simulink model "DeratingControl"  (R2021b)
settings: Solver=VariableStepAuto  StartTime=0.0  StopTime=1  FixedStep=Ts  RelTol=1e-3
model workspace (MAT data in the model file):
  df = Simulink.Parameter
  df.Value = 0.9
  df.DataType = 'auto'
  df.Complexity = 'real'
  df.Dimensions = [1 1]
undefined symbols (not defined in the file): const_facInvTempDera, const_facMotTempDera, const_facPwrDera, const_SCD_tqDeraGenOvrd_C, const_stDera, const_tqBattDeraGenLim, const_tqBattDeraMotLim, const_tqDeraGen, const_tqDeraMot, const_tqDeraMotOvrd_C, const_tqEmMaxNp1, const_tqInvTempDeraMax, const_tqInvTempDeraMin, const_tqMotTempDeraMax, const_tqMotTempDeraMin, const_tqSpLim, const_tqSpLimMax, const_tqSpLimMin, const_tqTqReq
libraries: hdlsllib x10
settings Model: PacingRate=0.350000  Creator=win  LastModifiedBy=win

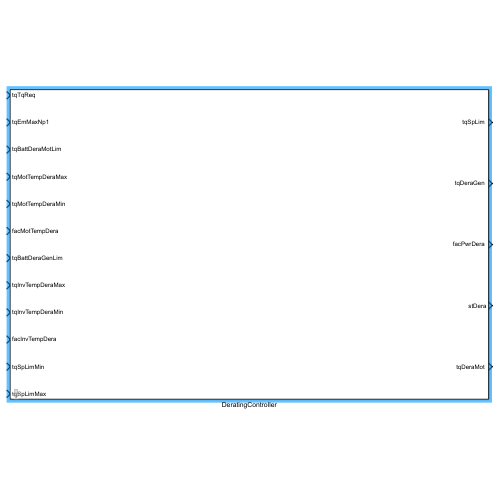
[thumbnail: Simulink's stored preview of the top-level diagram]
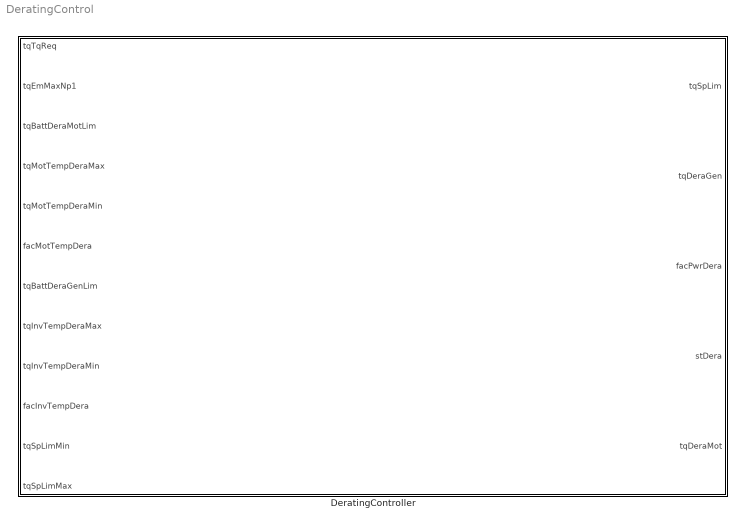
== system DeratingControl ==
  DeratingController : Subsystem  Description=Torque setpoint limit maximum value  mask{facGrdLimrUlim_C=5000, facGrdLimrLlim_C=-5000, bDeraMotOvrdActv_C=off, tqDeraMotOvrd_C=0, bDeraGenOvrdActv_C=off, SCD_tqDeraGenOvrd_C=0}
      mask prompts: facGrdLimrUlim_C "Gradient limiter upper factor"; facGrdLimrLlim_C "Gradient limiter lower factor"; bDeraMotOvrdActv_C "Motor mode derating override active"; tqDeraMotOvrd_C "Motor mode derating override torque"; bDeraGenOvrdActv_C "Generator mode derating override active"; SCD_tqDeraGenOvrd_C "Generator mode derating override torque"

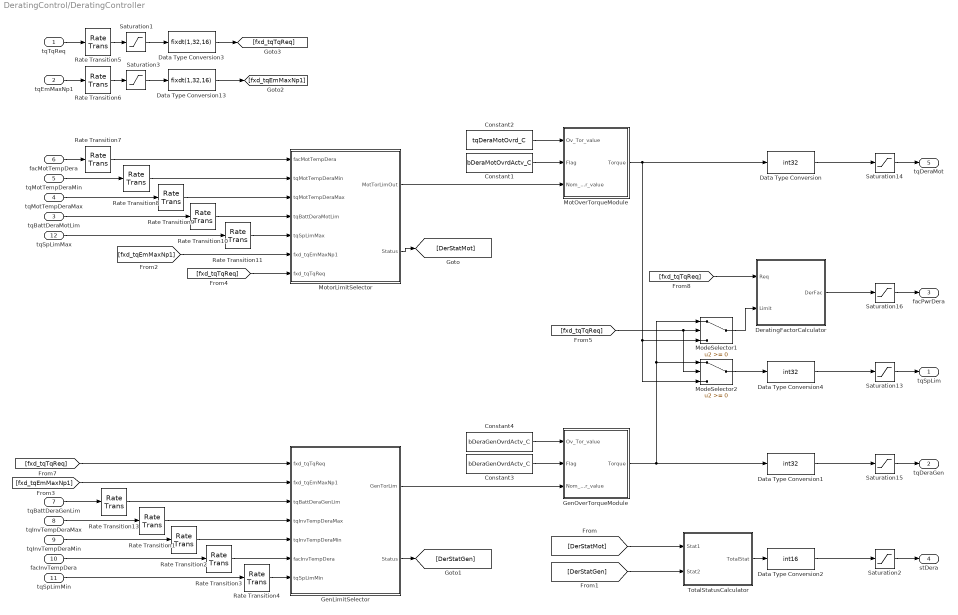
== system DeratingControl/DeratingController ==
  tqTqReq : Inport  Description=Torque request  OutMin=const_tqTqReq(1)  OutMax=const_tqTqReq(2)  OutDataTypeStr=int32
  tqEmMaxNp1 : Inport  Description=EM Maximum torque N+1 step  Port=2  OutMin=const_tqEmMaxNp1(1)  OutMax=const_tqEmMaxNp1(2)  OutDataTypeStr=int32
  tqBattDeraMotLim : Inport  Description=Derated motor mode torque output according to battery limits  Port=3  OutMin=const_tqBattDeraMotLim(1)  OutMax=const_tqBattDeraMotLim(2)  OutDataTypeStr=int32
  tqMotTempDeraMax : Inport  Description=Derated torque maximum value according to motor temperature  Port=4  OutMin=const_tqMotTempDeraMax(1)  OutMax=const_tqMotTempDeraMax(2)  OutDataTypeStr=int32
  tqMotTempDeraMin : Inport  Description=Derated torque minimum value according to motor temperature  Port=5  OutMin=const_tqMotTempDeraMin(1)  OutMax=const_tqMotTempDeraMin(2)  OutDataTypeStr=int32
  facMotTempDera : Inport  Description=Torque derating factor according to motor temperature  Port=6  OutMin=const_facMotTempDera(1)  OutMax=const_facMotTempDera(2)  OutDataTypeStr=int32
  tqBattDeraGenLim : Inport  Description=Derated generator mode torque output according to battery limits  Port=7  OutMin=const_tqBattDeraGenLim(1)  OutMax=const_tqBattDeraGenLim(2)  OutDataTypeStr=int32
  tqInvTempDeraMax : Inport  Description=Derated torque maximum value according to inverter temperature  Port=8  OutMin=const_tqInvTempDeraMax(1)  OutMax=const_tqInvTempDeraMax(2)  OutDataTypeStr=int32
  tqInvTempDeraMin : Inport  Description=Derated torque minimum value according to inverter temperature  Port=9  OutMin=const_tqInvTempDeraMin(1)  OutMax=const_tqInvTempDeraMin(2)  OutDataTypeStr=int32
  facInvTempDera : Inport  Description=Torque derating factor according to inverter temperature  Port=10  OutMin=const_facInvTempDera(1)  OutMax=const_facInvTempDera(2)  OutDataTypeStr=int32
  tqSpLimMin : Inport  Description=Torque setpoint limit minimum value  Port=11  OutMin=const_tqSpLimMin(1)  OutMax=const_tqSpLimMin(2)  OutDataTypeStr=int32
  tqSpLimMax : Inport  Description=Torque setpoint limit maximum value  Port=12  OutMin=const_tqSpLimMax(1)  OutMax=const_tqSpLimMax(2)  OutDataTypeStr=int32
  Constant1 : Constant  Value=bDeraMotOvrdActv_C
  Constant2 : Constant  Value=tqDeraMotOvrd_C
  Constant3 : Constant  Value=bDeraGenOvrdActv_C
  Constant4 : Constant  Value=bDeraGenOvrdActv_C
  Data Type Conversion : DataTypeConversion  OutDataTypeStr=int32
  Data Type Conversion1 : DataTypeConversion  OutDataTypeStr=int32
  Data Type Conversion13 : DataTypeConversion  OutDataTypeStr=fixdt(1,32,16)
  Data Type Conversion2 : DataTypeConversion  OutDataTypeStr=int16
  Data Type Conversion3 : DataTypeConversion  OutDataTypeStr=fixdt(1,32,16)
  Data Type Conversion4 : DataTypeConversion  OutDataTypeStr=int32
  DeratingFactorCalculator : Subsystem
  GenLimitSelector : Subsystem
  GenOverTorqueModule : Subsystem
  ModeSelector1 : Switch
  ModeSelector2 : Switch
  MotOverTorqueModule : Subsystem
  MotorLimitSelector : Subsystem
  Rate Transition{1..11,13} (12 alike) : RateTransition  OutPortSampleTime=Ts
  Saturation1 : Saturate  UpperLimit=const_tqTqReq(2)  LowerLimit=const_tqTqReq(1)
  Saturation13 : Saturate  UpperLimit=const_tqSpLim(2)  LowerLimit=const_tqSpLim(1)  OutDataTypeStr=int32
  Saturation14 : Saturate  UpperLimit=const_tqDeraMot(2)  LowerLimit=const_tqDeraMot(1)
  Saturation15 : Saturate  UpperLimit=const_tqDeraGen(2)  LowerLimit=const_tqDeraGen(1)
  Saturation16 : Saturate  UpperLimit=const_facPwrDera(2)  LowerLimit=const_facPwrDera(1)
  Saturation2 : Saturate  UpperLimit=const_stDera(2)  LowerLimit=const_stDera(1)  OutDataTypeStr=int32
  Saturation3 : Saturate  UpperLimit=const_tqEmMaxNp1(2)  LowerLimit=const_tqEmMaxNp1(1)
  TotalStatusCalculator : Subsystem
  "tqSpLim " : Outport  Description=Limited torque setpoint  OutMin=const_tqSpLim(1)  OutMax=const_tqSpLim(2)
  "tqDeraGen " : Outport  Description=Derated torque for generator mode  Port=2  OutMin=const_tqDeraGen(1)  OutMax=const_tqDeraGen(2)
  "facPwrDera " : Outport  Description=Power derating factor  Port=3  OutMin=const_facPwrDera(1)  OutMax=const_facPwrDera(2)
  stDera : Outport  Description=Derating status  Port=4
  "tqDeraMot " : Outport  Description=Derated torque for motor mode  Port=5
  wires:
  Saturation13/1 -> "tqSpLim "/1
  Saturation16/1 -> "facPwrDera "/1
  facMotTempDera/1 -> Rate Transition7/1
  tqMotTempDeraMin/1 -> Rate Transition8/1
  tqMotTempDeraMax/1 -> Rate Transition9/1
  tqBattDeraMotLim/1 -> Rate Transition10/1
  tqBattDeraGenLim/1 -> Rate Transition13/1
  tqInvTempDeraMax/1 -> Rate Transition1/1
  tqInvTempDeraMin/1 -> Rate Transition2/1
  facInvTempDera/1 -> Rate Transition3/1
  Constant4/1 -> GenOverTorqueModule/1(Ov_Tor_value)
  Constant3/1 -> GenOverTorqueModule/2(Flag)
  Constant2/1 -> MotOverTorqueModule/1(Ov_Tor_value)
  Constant1/1 -> MotOverTorqueModule/2(Flag)
  MotorLimitSelector/1(MotTorLimOut) -> MotOverTorqueModule/3(Nom_Tor_value)
  GenLimitSelector/1(GenTorLim) -> GenOverTorqueModule/3(Nom_Tor_value)
  Saturation15/1 -> "tqDeraGen "/1
  MotorLimitSelector/2(Status) -> [DerStatMot]
  GenOverTorqueModule/1(Torque) -> ModeSelector1/1, ModeSelector2/1, Data Type Conversion1/1
  GenLimitSelector/2(Status) -> [DerStatGen]
  [DerStatMot] -> TotalStatusCalculator/1(Stat1)
  [DerStatGen] -> TotalStatusCalculator/2(Stat2)
  Saturation2/1 -> stDera/1
  MotOverTorqueModule/1(Torque) -> ModeSelector2/3, ModeSelector1/3, Data Type Conversion/1
  tqSpLimMin/1 -> Rate Transition4/1
  tqSpLimMax/1 -> Rate Transition11/1
  ModeSelector2/1 -> Data Type Conversion4/1
  Saturation1/1 -> Data Type Conversion3/1
  Saturation3/1 -> Data Type Conversion13/1
  tqTqReq/1 -> Rate Transition5/1
  tqEmMaxNp1/1 -> Rate Transition6/1
  Rate Transition13/1 -> GenLimitSelector/3(tqBattDeraGenLim)
  Rate Transition1/1 -> GenLimitSelector/4(tqInvTempDeraMax)
  Rate Transition2/1 -> GenLimitSelector/5(tqInvTempDeraMin)
  Rate Transition3/1 -> GenLimitSelector/6("facInvTempDera ")
  Rate Transition4/1 -> GenLimitSelector/7("tqSpLimMin ")
  Rate Transition6/1 -> Saturation3/1
  Rate Transition5/1 -> Saturation1/1
  Rate Transition7/1 -> MotorLimitSelector/1("facMotTempDera ")
  Rate Transition8/1 -> MotorLimitSelector/2("tqMotTempDeraMin ")
  Rate Transition9/1 -> MotorLimitSelector/3("tqMotTempDeraMax ")
  Rate Transition10/1 -> MotorLimitSelector/4(tqBattDeraMotLim)
  Rate Transition11/1 -> MotorLimitSelector/5("tqSpLimMax ")
  Data Type Conversion13/1 -> [fxd_tqEmMaxNp1]
  [fxd_tqEmMaxNp1] -> MotorLimitSelector/6(fxd_tqEmMaxNp1)
  [fxd_tqEmMaxNp1] -> GenLimitSelector/2(fxd_tqEmMaxNp1)
  [fxd_tqTqReq] -> MotorLimitSelector/7(fxd_tqTqReq)
  Data Type Conversion3/1 -> [fxd_tqTqReq]
  [fxd_tqTqReq] -> ModeSelector2/2, ModeSelector1/2
  [fxd_tqTqReq] -> GenLimitSelector/1(fxd_tqTqReq)
  Data Type Conversion/1 -> Saturation14/1
  Saturation14/1 -> "tqDeraMot "/1
  Data Type Conversion1/1 -> Saturation15/1
  [fxd_tqTqReq] -> DeratingFactorCalculator/1(Req)
  ModeSelector1/1 -> DeratingFactorCalculator/2(Limit)
  DeratingFactorCalculator/1(DerFac) -> Saturation16/1
  Data Type Conversion4/1 -> Saturation13/1
  TotalStatusCalculator/1(TotalStat) -> Data Type Conversion2/1
  Data Type Conversion2/1 -> Saturation2/1

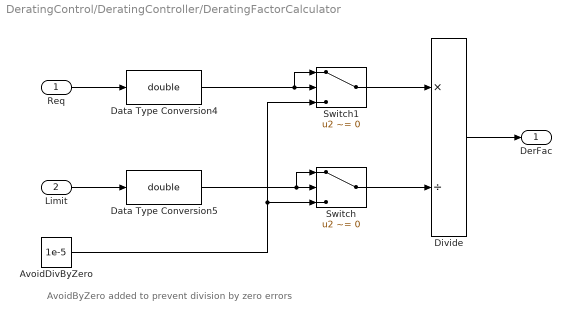
== system DeratingControl/DeratingController/DeratingFactorCalculator ==
  note: AvoidByZero added to prevent division by zero errors
  Req : Inport
  Limit : Inport  Port=2
  AvoidDivByZero : Constant  Value=1e-5  OutDataTypeStr=Inherit: Inherit via back propagation
  Data Type Conversion4 : DataTypeConversion  OutDataTypeStr=double
  Data Type Conversion5 : DataTypeConversion  OutDataTypeStr=double
  Divide : Product  Inputs=*/
  Switch : Switch  Criteria=u2 ~= 0  Threshold=1e-4
  Switch1 : Switch  Criteria=u2 ~= 0  Threshold=1e-4
  DerFac : Outport
  wires:
  Divide/1 -> DerFac/1
  Req/1 -> Data Type Conversion4/1
  Limit/1 -> Data Type Conversion5/1
  Data Type Conversion5/1 -> Switch/2, Switch/1
  Switch/1 -> Divide/2
  AvoidDivByZero/1 -> Switch/3, Switch1/3
  Switch1/1 -> Divide/1
  Data Type Conversion4/1 -> Switch1/2, Switch1/1

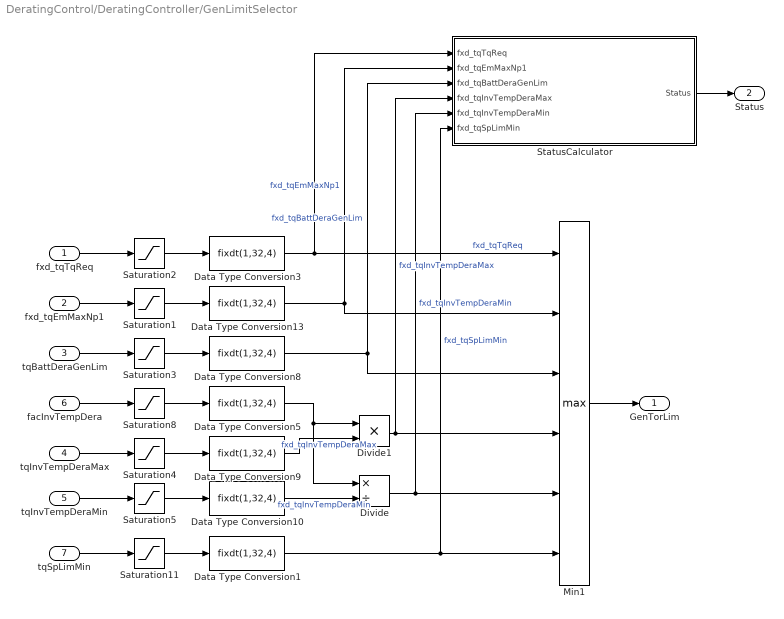
== system DeratingControl/DeratingController/GenLimitSelector ==
  fxd_tqTqReq : Inport
  fxd_tqEmMaxNp1 : Inport  Port=2
  tqBattDeraGenLim : Inport  Description=Derated generator mode torque output according to battery limits  Port=3  OutMin=const_tqBattDeraGenLim(1)  OutMax=const_tqBattDeraGenLim(2)  OutDataTypeStr=int32
  tqInvTempDeraMax : Inport  Description=Derated torque maximum value according to inverter temperature  Port=4  OutMin=const_tqInvTempDeraMax(1)  OutMax=const_tqInvTempDeraMax(2)  OutDataTypeStr=int32
  tqInvTempDeraMin : Inport  Description=Derated torque minimum value according to inverter temperature  Port=5  OutMin=const_tqInvTempDeraMin(1)  OutMax=const_tqInvTempDeraMin(2)  OutDataTypeStr=int32
  "facInvTempDera " : Inport  Description=Torque derating factor according to inverter temperature  Port=6  OutMin=const_facInvTempDera(1)  OutMax=const_facInvTempDera(2)  OutDataTypeStr=int32
  "tqSpLimMin " : Inport  Port=7
  Data Type Conversion{1,3,5,8..10,13} (7 alike) : DataTypeConversion  OutDataTypeStr=fixdt(1,32,4)
  Divide : Product  Inputs=*/
  Divide1 : Product  Inputs=**
  Min1 : MinMax  Function=max  Inputs=6
  Saturation1 : Saturate  UpperLimit=const_tqEmMaxNp1(2)  LowerLimit=const_tqEmMaxNp1(1)  OutDataTypeStr=double
  Saturation11 : Saturate  UpperLimit=const_tqSpLimMin(2)  LowerLimit=const_tqSpLimMin(1)  OutDataTypeStr=int32
  Saturation2 : Saturate  UpperLimit=const_tqTqReq(2)  LowerLimit=const_tqTqReq(1)  OutDataTypeStr=fixdt(1,32,12)
  Saturation3 : Saturate  UpperLimit=const_tqBattDeraGenLim(2)  LowerLimit=const_tqBattDeraGenLim(1)
  Saturation4 : Saturate  UpperLimit=const_tqInvTempDeraMax(2)  LowerLimit=const_tqInvTempDeraMax(1)  OutDataTypeStr=int32
  Saturation5 : Saturate  UpperLimit=const_tqInvTempDeraMin(2)  LowerLimit=const_tqInvTempDeraMin(1)  OutDataTypeStr=int32
  Saturation8 : Saturate  UpperLimit=1  LowerLimit=0  OutDataTypeStr=int32
  StatusCalculator : Subsystem
  GenTorLim : Outport
  Status : Outport  Port=2
  wires:
  Divide1/1 -> StatusCalculator/4(fxd_tqInvTempDeraMax), Min1/4  "fxd_tqInvTempDeraMax"
  Data Type Conversion8/1 -> Min1/3, StatusCalculator/3(fxd_tqBattDeraGenLim)  "fxd_tqBattDeraGenLim"
  Divide/1 -> StatusCalculator/5(fxd_tqInvTempDeraMin), Min1/5  "fxd_tqInvTempDeraMin"
  Saturation8/1 -> Data Type Conversion5/1
  Saturation4/1 -> Data Type Conversion9/1
  fxd_tqEmMaxNp1/1 -> Saturation1/1
  fxd_tqTqReq/1 -> Saturation2/1
  Saturation3/1 -> Data Type Conversion8/1
  Min1/1 -> GenTorLim/1
  "facInvTempDera "/1 -> Saturation8/1
  tqBattDeraGenLim/1 -> Saturation3/1
  tqInvTempDeraMax/1 -> Saturation4/1
  Saturation5/1 -> Data Type Conversion10/1
  tqInvTempDeraMin/1 -> Saturation5/1
  StatusCalculator/1(Status) -> Status/1
  Data Type Conversion13/1 -> Min1/2, StatusCalculator/2(fxd_tqEmMaxNp1)  "fxd_tqEmMaxNp1"
  Saturation1/1 -> Data Type Conversion13/1
  Data Type Conversion3/1 -> StatusCalculator/1(fxd_tqTqReq), Min1/1  "fxd_tqTqReq"
  Saturation2/1 -> Data Type Conversion3/1
  Saturation11/1 -> Data Type Conversion1/1
  Data Type Conversion1/1 -> Min1/6, StatusCalculator/6(fxd_tqSpLimMin)  "fxd_tqSpLimMin"
  "tqSpLimMin "/1 -> Saturation11/1
  Data Type Conversion10/1 -> Divide/2  "fxd_tqInvTempDeraMin"
  Data Type Conversion5/1 -> Divide/1, Divide1/1
  Data Type Conversion9/1 -> Divide1/2  "fxd_tqInvTempDeraMax"

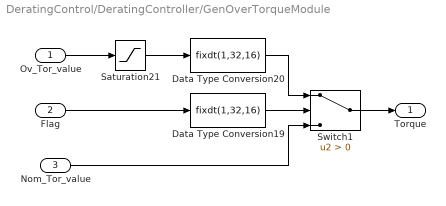
== system DeratingControl/DeratingController/GenOverTorqueModule ==
  Ov_Tor_value : Inport
  Flag : Inport  Port=2
  Nom_Tor_value : Inport  Port=3
  Data Type Conversion19 : DataTypeConversion  OutDataTypeStr=fixdt(1,32,16)
  Data Type Conversion20 : DataTypeConversion  OutDataTypeStr=fixdt(1,32,16)
  Saturation21 : Saturate  UpperLimit=const_SCD_tqDeraGenOvrd_C(2)  LowerLimit=const_SCD_tqDeraGenOvrd_C(1)  OutDataTypeStr=int32
  Switch1 : Switch  Criteria=u2 > Threshold  OutDataTypeStr=fixdt(1,32,16)
  Torque : Outport
  wires:
  Flag/1 -> Data Type Conversion19/1
  Saturation21/1 -> Data Type Conversion20/1
  Ov_Tor_value/1 -> Saturation21/1
  Data Type Conversion20/1 -> Switch1/1
  Data Type Conversion19/1 -> Switch1/2
  Switch1/1 -> Torque/1
  Nom_Tor_value/1 -> Switch1/3

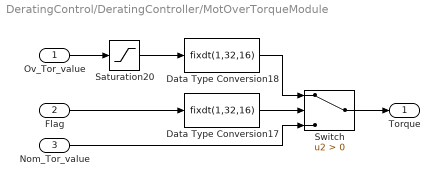
== system DeratingControl/DeratingController/MotOverTorqueModule ==
  Ov_Tor_value : Inport
  Flag : Inport  Port=2
  Nom_Tor_value : Inport  Port=3
  Data Type Conversion17 : DataTypeConversion  OutDataTypeStr=fixdt(1,32,16)
  Data Type Conversion18 : DataTypeConversion  OutDataTypeStr=fixdt(1,32,16)
  Saturation20 : Saturate  UpperLimit=const_tqDeraMotOvrd_C(2)  LowerLimit=const_tqDeraMotOvrd_C(1)  OutDataTypeStr=int32
  Switch : Switch  Criteria=u2 > Threshold  OutDataTypeStr=fixdt(1,32,16)
  Torque : Outport
  wires:
  Ov_Tor_value/1 -> Saturation20/1
  Saturation20/1 -> Data Type Conversion18/1
  Switch/1 -> Torque/1
  Data Type Conversion17/1 -> Switch/2
  Nom_Tor_value/1 -> Switch/3
  Data Type Conversion18/1 -> Switch/1
  Flag/1 -> Data Type Conversion17/1

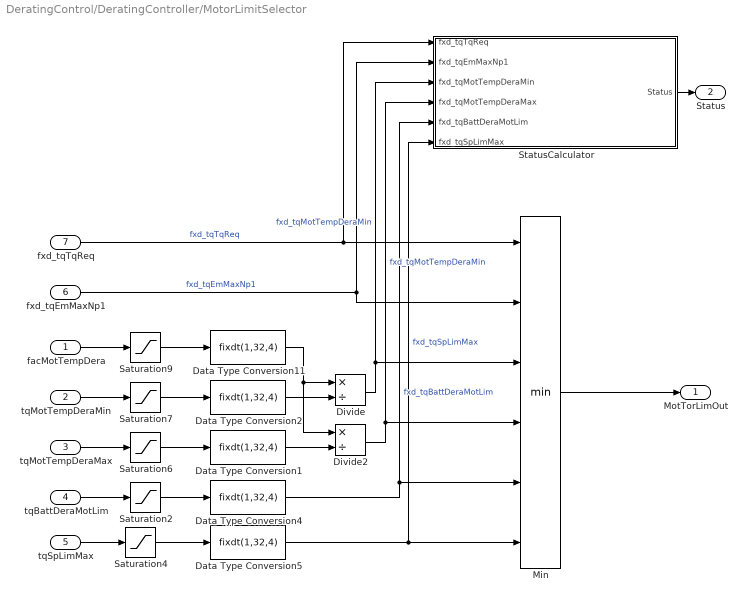
== system DeratingControl/DeratingController/MotorLimitSelector ==
  "facMotTempDera " : Inport  Description=Torque derating factor according to motor temperature  OutMin=const_facMotTempDera(1)  OutMax=const_facMotTempDera(2)  OutDataTypeStr=int32
  "tqMotTempDeraMin " : Inport  Description=Derated torque minimum value according to motor temperature  Port=2  OutMin=const_tqMotTempDeraMin(1)  OutMax=const_tqMotTempDeraMin(2)  OutDataTypeStr=int32
  "tqMotTempDeraMax " : Inport  Description=Derated torque maximum value according to motor temperature  Port=3  OutMin=const_tqMotTempDeraMax(1)  OutMax=const_tqMotTempDeraMax(2)  OutDataTypeStr=int32
  tqBattDeraMotLim : Inport  Description=Derated motor mode torque output according to battery limits  Port=4  OutMin=const_tqBattDeraMotLim(1)  OutMax=const_tqBattDeraMotLim(2)  OutDataTypeStr=int32
  "tqSpLimMax " : Inport  Port=5
  fxd_tqEmMaxNp1 : Inport  Port=6
  fxd_tqTqReq : Inport  Port=7
  Data Type Conversion{1..2,4..5,11} (5 alike) : DataTypeConversion  OutDataTypeStr=fixdt(1,32,4)
  Divide : Product  Inputs=*/
  Divide2 : Product  Inputs=*/
  Min : MinMax  Inputs=6
  Saturation2 : Saturate  UpperLimit=const_tqBattDeraMotLim(2)  LowerLimit=const_tqBattDeraMotLim(1)
  Saturation4 : Saturate  UpperLimit=const_tqSpLimMax(2)  LowerLimit=const_tqSpLimMax(1)
  Saturation6 : Saturate  UpperLimit=const_tqMotTempDeraMax(2)  LowerLimit=const_tqMotTempDeraMax(1)  OutDataTypeStr=int32
  Saturation7 : Saturate  UpperLimit=const_tqMotTempDeraMin(2)  LowerLimit=const_tqMotTempDeraMin(1)  OutDataTypeStr=int32
  Saturation9 : Saturate  UpperLimit=const_facMotTempDera(2)  LowerLimit=const_facMotTempDera(1)  OutDataTypeStr=int32
  StatusCalculator : Subsystem
  MotTorLimOut : Outport
  Status : Outport  Port=2
  wires:
  Saturation7/1 -> Data Type Conversion2/1
  Saturation9/1 -> Data Type Conversion11/1
  tqBattDeraMotLim/1 -> Saturation2/1
  Data Type Conversion2/1 -> Divide/2
  "tqMotTempDeraMax "/1 -> Saturation6/1
  Saturation2/1 -> Data Type Conversion4/1
  Min/1 -> MotTorLimOut/1
  Saturation6/1 -> Data Type Conversion1/1
  Data Type Conversion4/1 -> Min/5, StatusCalculator/5(fxd_tqBattDeraMotLim)  "fxd_tqBattDeraMotLim"
  "facMotTempDera "/1 -> Saturation9/1
  "tqMotTempDeraMin "/1 -> Saturation7/1
  Data Type Conversion11/1 -> Divide2/1, Divide/1
  StatusCalculator/1(Status) -> Status/1
  fxd_tqTqReq/1 -> StatusCalculator/1(fxd_tqTqReq), Min/1  "fxd_tqTqReq"
  fxd_tqEmMaxNp1/1 -> StatusCalculator/2(fxd_tqEmMaxNp1), Min/2  "fxd_tqEmMaxNp1"
  "tqSpLimMax "/1 -> Saturation4/1
  Saturation4/1 -> Data Type Conversion5/1
  Data Type Conversion5/1 -> StatusCalculator/6(fxd_tqSpLimMax), Min/6  "fxd_tqSpLimMax"
  Divide/1 -> Min/3, StatusCalculator/3(fxd_tqMotTempDeraMin)  "fxd_tqMotTempDeraMin"
  Data Type Conversion1/1 -> Divide2/2
  Divide2/1 -> Min/4, StatusCalculator/4(fxd_tqMotTempDeraMax)  "fxd_tqMotTempDeraMin"

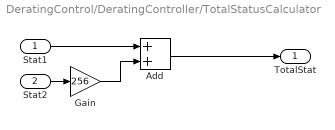
== system DeratingControl/DeratingController/TotalStatusCalculator ==
  Stat1 : Inport
  Stat2 : Inport  Port=2
  Add : Sum
  Gain : Gain  Gain=256
  TotalStat : Outport
  wires:
  Stat1/1 -> Add/1
  Gain/1 -> Add/2
  Stat2/1 -> Gain/1
  Add/1 -> TotalStat/1

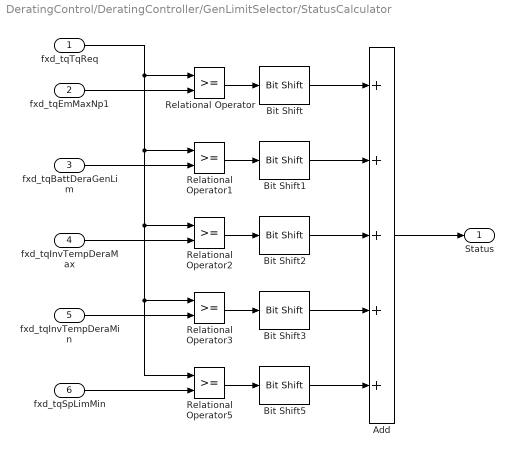
== system DeratingControl/DeratingController/GenLimitSelector/StatusCalculator ==
  fxd_tqTqReq : Inport
  fxd_tqEmMaxNp1 : Inport  Port=2
  fxd_tqBattDeraGenLim : Inport  Port=3
  fxd_tqInvTempDeraMax : Inport  Port=4
  fxd_tqInvTempDeraMin : Inport  Port=5
  fxd_tqSpLimMin : Inport  Port=6
  Add : Sum  Inputs=+++++
  Bit Shift : hdlsllib/Logic and Bit Operations/Bit Shift  mode=Shift Left Logical  N=0
  Bit Shift1 : hdlsllib/Logic and Bit Operations/Bit Shift  mode=Shift Left Logical  N=1
  Bit Shift2 : hdlsllib/Logic and Bit Operations/Bit Shift  mode=Shift Left Logical  N=2
  Bit Shift3 : hdlsllib/Logic and Bit Operations/Bit Shift  mode=Shift Left Logical  N=3
  Bit Shift5 : hdlsllib/Logic and Bit Operations/Bit Shift  mode=Shift Left Logical  N=4
  Relational Operator{,1..3,5} (5 alike) : RelationalOperator  OutDataTypeStr=fixdt(1,16,0)  RndMeth=Simplest
  Status : Outport
  wires:
  fxd_tqTqReq/1 -> Relational Operator1/1, Relational Operator5/1, Relational Operator3/1, Relational Operator2/1, Relational Operator/1
  fxd_tqEmMaxNp1/1 -> Relational Operator/2
  Relational Operator/1 -> Bit Shift/1
  Add/1 -> Status/1
  Relational Operator1/1 -> Bit Shift1/1
  fxd_tqBattDeraGenLim/1 -> Relational Operator1/2
  Bit Shift1/1 -> Add/2
  Bit Shift/1 -> Add/1
  Relational Operator2/1 -> Bit Shift2/1
  Bit Shift2/1 -> Add/3
  fxd_tqInvTempDeraMax/1 -> Relational Operator2/2
  fxd_tqInvTempDeraMin/1 -> Relational Operator3/2
  Relational Operator3/1 -> Bit Shift3/1
  Bit Shift3/1 -> Add/4
  Bit Shift5/1 -> Add/5
  fxd_tqSpLimMin/1 -> Relational Operator5/2
  Relational Operator5/1 -> Bit Shift5/1

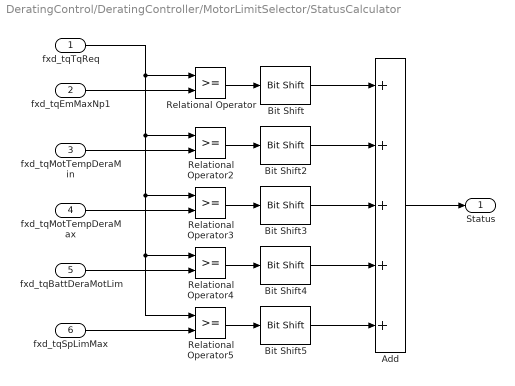
== system DeratingControl/DeratingController/MotorLimitSelector/StatusCalculator ==
  fxd_tqTqReq : Inport
  fxd_tqEmMaxNp1 : Inport  Port=2
  fxd_tqMotTempDeraMin : Inport  Port=3
  fxd_tqMotTempDeraMax : Inport  Port=4
  fxd_tqBattDeraMotLim : Inport  Port=5
  fxd_tqSpLimMax : Inport  Port=6
  Add : Sum  Inputs=+++++
  Bit Shift : hdlsllib/Logic and Bit Operations/Bit Shift  mode=Shift Left Logical  N=0
  Bit Shift2 : hdlsllib/Logic and Bit Operations/Bit Shift  mode=Shift Left Logical  N=1
  Bit Shift3 : hdlsllib/Logic and Bit Operations/Bit Shift  mode=Shift Left Logical  N=2
  Bit Shift4 : hdlsllib/Logic and Bit Operations/Bit Shift  mode=Shift Left Logical  N=3
  Bit Shift5 : hdlsllib/Logic and Bit Operations/Bit Shift  mode=Shift Left Logical  N=4
  Relational Operator{,2..5} (5 alike) : RelationalOperator  OutDataTypeStr=fixdt(1,16,0)  RndMeth=Simplest
  Status : Outport
  wires:
  fxd_tqTqReq/1 -> Relational Operator4/1, Relational Operator5/1, Relational Operator3/1, Relational Operator2/1, Relational Operator/1
  Relational Operator/1 -> Bit Shift/1
  Add/1 -> Status/1
  Bit Shift/1 -> Add/1
  Relational Operator2/1 -> Bit Shift2/1
  Bit Shift2/1 -> Add/2
  Relational Operator3/1 -> Bit Shift3/1
  Bit Shift3/1 -> Add/3
  Bit Shift4/1 -> Add/4
  Relational Operator4/1 -> Bit Shift4/1
  fxd_tqEmMaxNp1/1 -> Relational Operator/2
  fxd_tqMotTempDeraMin/1 -> Relational Operator2/2
  fxd_tqMotTempDeraMax/1 -> Relational Operator3/2
  Relational Operator5/1 -> Bit Shift5/1
  Bit Shift5/1 -> Add/5
  fxd_tqBattDeraMotLim/1 -> Relational Operator4/2
  fxd_tqSpLimMax/1 -> Relational Operator5/2
